simulink model "rtmc_x"  (R2014b)
settings: Solver=ode45  StartTime=0.0  StopTime=500  RelTol=1e-3
settings Model: Creator=mkatliar  LastModifiedBy=mkatliar

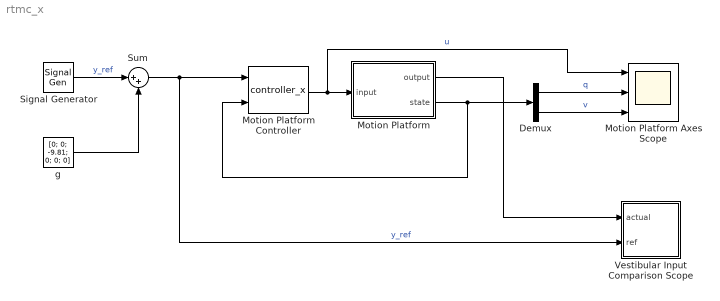
== system rtmc_x ==
  Demux : Demux  Outputs=[1; 1]
  Motion Platform : Subsystem
  Motion Platform Axes Scope : Scope  NumInputPorts=3
      settings: TimeRange=10  YMin=-1~0~-0.2  YMax=1~0.8~0.4  ScrollMode=on
  Motion Platform Controller : S-Function  FunctionName=controller_x  EnableBusSupport=off
  Signal Generator : SignalGenerator  Amplitude=[1, 0, 0, 0, 0, 0]
  Sum : Sum  Inputs=|++
  Vestibular Input Comparison Scope : Subsystem
  g : Constant  Value=[0; 0; -9.81; 0; 0; 0]
  wires:
  Motion Platform Controller/1 -> Motion Platform Axes Scope/1, Motion Platform/1(input)  "u"
  Sum/1 -> Motion Platform Controller/1, Vestibular Input Comparison Scope/2(ref)  "y_ref"
  g/1 -> Sum/2
  Signal Generator/1 -> Sum/1  "y_ref"
  Demux/1 -> Motion Platform Axes Scope/2  "q"
  Motion Platform/1(output) -> Vestibular Input Comparison Scope/1(actual)
  Motion Platform/2(state) -> Demux/1, Motion Platform Controller/2
  Demux/2 -> Motion Platform Axes Scope/3  "v"

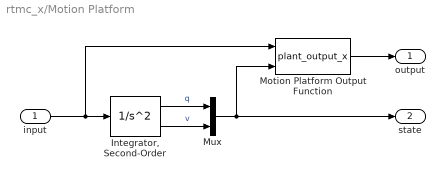
== system rtmc_x/Motion Platform ==
  input : Inport
  "Integrator, Second-Order" : SecondOrderIntegrator  ICX=0  ICDXDT=0
  Motion Platform Output Function : S-Function  FunctionName=plant_output_x  EnableBusSupport=off
  Mux : Mux  Inputs=2
  output : Outport
  state : Outport  Port=2
  wires:
  "Integrator, Second-Order"/1 -> Mux/1  "q"
  "Integrator, Second-Order"/2 -> Mux/2  "v"
  Mux/1 -> state/1, Motion Platform Output Function/2
  Motion Platform Output Function/1 -> output/1
  input/1 -> "Integrator, Second-Order"/1, Motion Platform Output Function/1

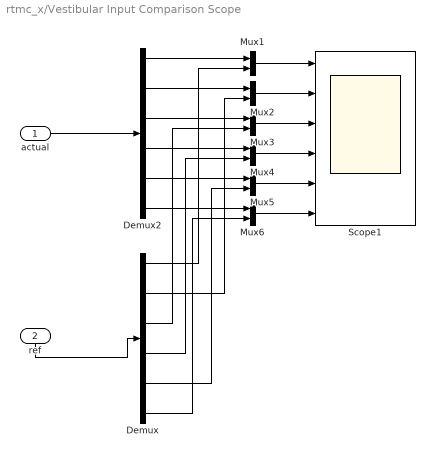
== system rtmc_x/Vestibular Input Comparison Scope ==
  actual : Inport
  ref : Inport  Port=2
  Demux : Demux  Outputs=6
  Demux2 : Demux  Outputs=6
  Mux{1..6} (6 alike) : Mux  Inputs=2
  Scope1 : Scope  NumInputPorts=6
      settings: TimeRange=10  YMin=-1~-1~-10~-1~-1~-1  YMax=1~1~0~1~1~1
  wires:
  Demux/4 -> Mux4/2
  Demux2/1 -> Mux1/1
  Demux/2 -> Mux2/2
  Demux/5 -> Mux5/2
  Mux2/1 -> Scope1/2
  Demux2/3 -> Mux3/1
  Demux2/2 -> Mux2/1
  Demux/1 -> Mux1/2
  Demux/6 -> Mux6/2
  Demux2/4 -> Mux4/1
  Demux/3 -> Mux3/2
  Demux2/6 -> Mux6/1
  Demux2/5 -> Mux5/1
  Mux1/1 -> Scope1/1
  Mux3/1 -> Scope1/3
  Mux4/1 -> Scope1/4
  Mux5/1 -> Scope1/5
  Mux6/1 -> Scope1/6
  actual/1 -> Demux2/1
  ref/1 -> Demux/1
